simulink model "CompassDriver"  (Simulink 7.0)
settings: Solver=ode45  StartTime=0.0  StopTime=10.0  RelTol=1e-3
settings Model: Creator=volgy  LastModifiedBy=volgy

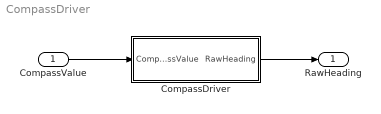
== system CompassDriver ==
  CompassValue : Inport  OutDataType=sfix(16)  OutScaling=2^0
  CompassDriver : Subsystem
  RawHeading : Outport  OutDataType=sfix(16)  OutScaling=2^0
  wires:
  CompassValue/1 -> CompassDriver/1(CompassValue)
  CompassDriver/1(RawHeading) -> RawHeading/1

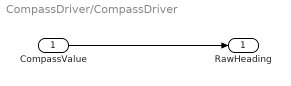
== system CompassDriver/CompassDriver ==
  CompassValue : Inport  OutDataType=sfix(16)  OutScaling=2^0
  RawHeading : Outport  OutDataType=sfix(16)  OutScaling=2^0
  wires:
  CompassValue/1 -> RawHeading/1
